simulink model "MyPowerSupply_RTW"  (R2022a)
settings: Solver=ode1  StartTime=0.0  StopTime=inf  FixedStep=0.0002  RelTol=1e-3
PreLoadFcn:
  | vehicle = 'Car'; if ~length(which('cmself')), cmenv; end
  | MyPowerSupply_RTW_bus
InitFcn:
  | vehicle = 'Car'; if ~length(which('cmself')), cmenv; end
  | MyPowerSupply_RTW_bus
libraries: CarMaker4SL x3, simulink x2, simulink_need_slupdate x1
Description:
  | CarMaker Plug-in Model Target
settings Model: ModifiedByFormat=IPG  Creator=IPG  LastModifiedBy=IPG
settings SolverCC: AlgebraicLoopSolver=TrustRegion
settings DebuggingCC: UnconnectedInputMsg=warning  UnconnectedOutputMsg=warning  UnconnectedLineMsg=warning  SFMachineParentedDataDiag=warning
settings RTWCC: Description=CarMaker Plug-in Model Target  SystemTargetFile=CarMaker.tlc  TemplateMakefile=CarMaker_unix-win64.tmf  DLArmComputeVersion=19.05
settings CodeAppCC: MaxIdLength=127
settings STFCustomTargetCC: TargetLangStandard=C99 (ISO)  CombineOutputUpdateFcns=on  CodeInterfacePackaging=Reusable function  GRTInterface=off  GenerateAllocFcn=on  SystemTargetFile=CarMaker.tlc
settings GRTTargetCC: ParMdlRefBuildCompliant=off  CompOptLevelCompliant=off  ConcurrentExecutionCompliant=off  MatFileLogging=off  CodeInterfacePackaging=Reusable function  CPPClassGenCompliant=off  GenerateAllocFcn=on  UseToolchainInfoCompliant=off

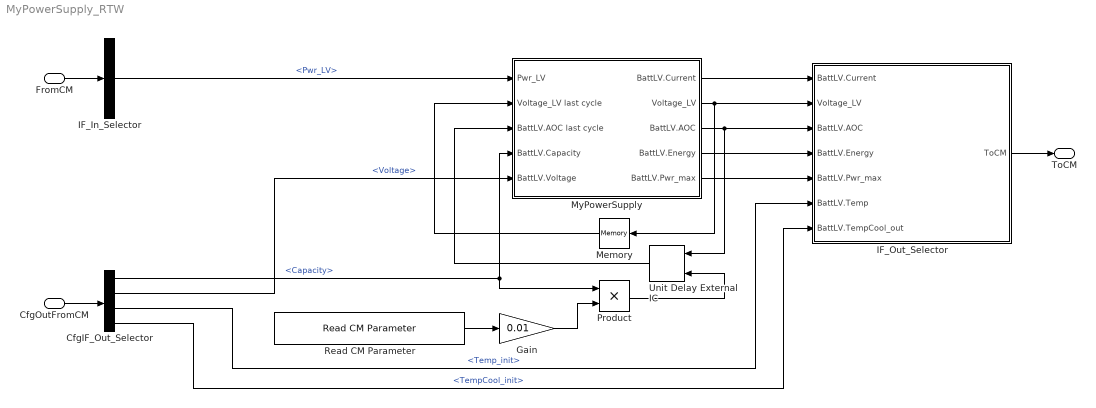
== system MyPowerSupply_RTW ==
  FromCM : Inport  OutDataTypeStr=Bus: cmPTPowerSupplyIn
  CfgOutFromCM : Inport  Port=2  OutDataTypeStr=Bus: cmPTPowerSupplyCfgOut
  CfgIF_Out_Selector : BusSelector  OutputSignals=BattLV.Capacity,BattLV.Voltage,BattLV.Temp_init,BattLV.TempCool_init
  Gain : Gain  Gain=0.01
  IF_In_Selector : BusSelector  OutputSignals=Pwr_LV
  IF_Out_Selector : Subsystem  mask(Signal Selection){}
      mask help: Signal Selection Block
      settings: OpenFcn=cmSignalSelect('SignalSelection_CB',gcb)
  Memory : Memory
  MyPowerSupply : Subsystem
  Product : Product  RndMeth=Zero
  Read CM Parameter : CarMaker4SL/Read CM Parameter  xfile_type=Vehicle  xfile_instance_vehicle=-  xfile_instance_trailer=1  xfile_instance_general=-  xfile_kind_vehicle=Vehicle  xfile_kind_trailer=Trailer  xfile_kind_general=SimParameters  xfile=Vehicle  xkey=PowerTrain.PowerSupply.BattLV.SOC  xnout=1  xdefaults=70.0  xmuxed=on  xstime=Continuous
      settings: SourceProductName=CarMaker4SL
  Unit Delay External IC : simulink_need_slupdate/Unit Delay External IC  tsamp=-1
      settings: SourceProductBaseCode=SL
  ToCM : Outport  OutDataTypeStr=Bus: cmPTPowerSupplyOut
  wires:
  Gain/1 -> Product/2
  CfgIF_Out_Selector/3 -> IF_Out_Selector/6(BattLV.Temp)  "<Temp_init>"
  MyPowerSupply/4(BattLV.Energy) -> IF_Out_Selector/4(BattLV.Energy)
  CfgIF_Out_Selector/1 -> Product/1, MyPowerSupply/4(BattLV.Capacity)  "<Capacity>"
  MyPowerSupply/3(BattLV.AOC) -> Unit Delay External IC/1, IF_Out_Selector/3(BattLV.AOC)
  Read CM Parameter/1 -> Gain/1
  IF_Out_Selector/1(ToCM) -> ToCM/1
  MyPowerSupply/1(BattLV.Current) -> IF_Out_Selector/1(BattLV.Current)
  CfgIF_Out_Selector/2 -> MyPowerSupply/5(BattLV.Voltage)  "<Voltage>"
  IF_In_Selector/1 -> MyPowerSupply/1(Pwr_LV)  "<Pwr_LV>"
  MyPowerSupply/5(BattLV.Pwr_max) -> IF_Out_Selector/5(BattLV.Pwr_max)
  CfgOutFromCM/1 -> CfgIF_Out_Selector/1
  MyPowerSupply/2(Voltage_LV) -> Memory/1, IF_Out_Selector/2(Voltage_LV)
  Memory/1 -> MyPowerSupply/2(Voltage_LV last cycle)
  CfgIF_Out_Selector/4 -> IF_Out_Selector/7(BattLV.TempCool_out)  "<TempCool_init>"
  Unit Delay External IC/1 -> MyPowerSupply/3(BattLV.AOC last cycle)
  FromCM/1 -> IF_In_Selector/1
  Product/1 -> Unit Delay External IC/2

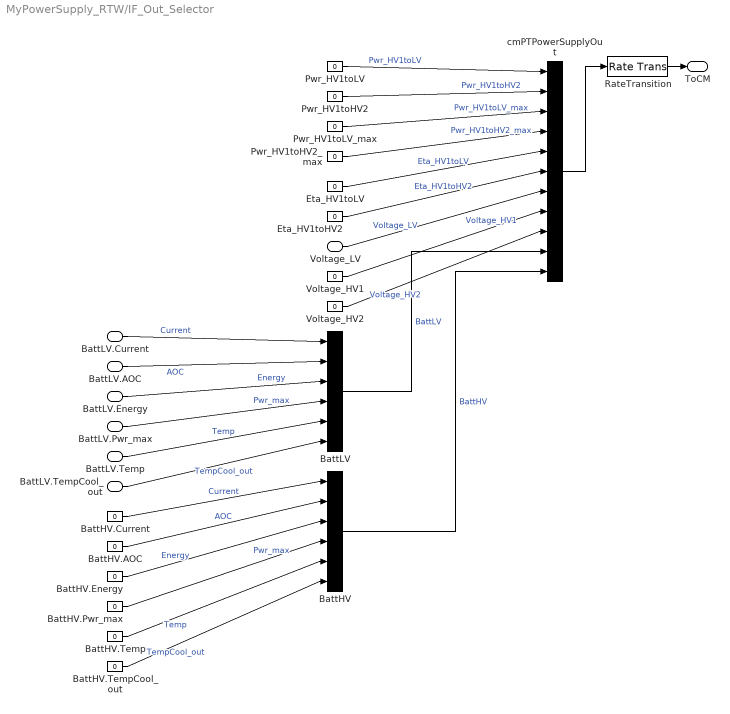
== system MyPowerSupply_RTW/IF_Out_Selector ==
  BattLV.Current : Inport
  Voltage_LV : Inport  Port=2
  BattLV.AOC : Inport  Port=3
  BattLV.Energy : Inport  Port=4
  BattLV.Pwr_max : Inport  Port=5
  BattLV.Temp : Inport  Port=6
  BattLV.TempCool_out : Inport  Port=7
  BattHV : BusCreator  Inputs=6
  BattHV.AOC : Constant  Value=0
  BattHV.Current : Constant  Value=0
  BattHV.Energy : Constant  Value=0
  BattHV.Pwr_max : Constant  Value=0
  BattHV.Temp : Constant  Value=0
  BattHV.TempCool_out : Constant  Value=0
  BattLV : BusCreator  Inputs=6
  Eta_HV1toHV2 : Constant  Value=0
  Eta_HV1toLV : Constant  Value=0
  Pwr_HV1toHV2 : Constant  Value=0
  Pwr_HV1toHV2_max : Constant  Value=0
  Pwr_HV1toLV : Constant  Value=0
  Pwr_HV1toLV_max : Constant  Value=0
  RateTransition : RateTransition  OutPortSampleTime=str2num(get_param(bdroot,'FixedStep'))
  Voltage_HV1 : Constant  Value=0
  Voltage_HV2 : Constant  Value=0
  cmPTPowerSupplyOut : BusCreator  Inputs=11
  ToCM : Outport
  wires:
  RateTransition/1 -> ToCM/1
  cmPTPowerSupplyOut/1 -> RateTransition/1
  Pwr_HV1toLV/1 -> cmPTPowerSupplyOut/1  "Pwr_HV1toLV"
  Pwr_HV1toHV2/1 -> cmPTPowerSupplyOut/2  "Pwr_HV1toHV2"
  Pwr_HV1toLV_max/1 -> cmPTPowerSupplyOut/3  "Pwr_HV1toLV_max"
  Pwr_HV1toHV2_max/1 -> cmPTPowerSupplyOut/4  "Pwr_HV1toHV2_max"
  Eta_HV1toLV/1 -> cmPTPowerSupplyOut/5  "Eta_HV1toLV"
  Eta_HV1toHV2/1 -> cmPTPowerSupplyOut/6  "Eta_HV1toHV2"
  Voltage_HV1/1 -> cmPTPowerSupplyOut/8  "Voltage_HV1"
  Voltage_HV2/1 -> cmPTPowerSupplyOut/9  "Voltage_HV2"
  BattLV/1 -> cmPTPowerSupplyOut/10  "BattLV"
  BattHV/1 -> cmPTPowerSupplyOut/11  "BattHV"
  BattHV.Current/1 -> BattHV/1  "Current"
  BattHV.AOC/1 -> BattHV/2  "AOC"
  BattHV.Energy/1 -> BattHV/3  "Energy"
  BattHV.Pwr_max/1 -> BattHV/4  "Pwr_max"
  BattHV.Temp/1 -> BattHV/5  "Temp"
  BattHV.TempCool_out/1 -> BattHV/6  "TempCool_out"
  BattLV.Current/1 -> BattLV/1  "Current"
  Voltage_LV/1 -> cmPTPowerSupplyOut/7  "Voltage_LV"
  BattLV.AOC/1 -> BattLV/2  "AOC"
  BattLV.Energy/1 -> BattLV/3  "Energy"
  BattLV.Pwr_max/1 -> BattLV/4  "Pwr_max"
  BattLV.Temp/1 -> BattLV/5  "Temp"
  BattLV.TempCool_out/1 -> BattLV/6  "TempCool_out"

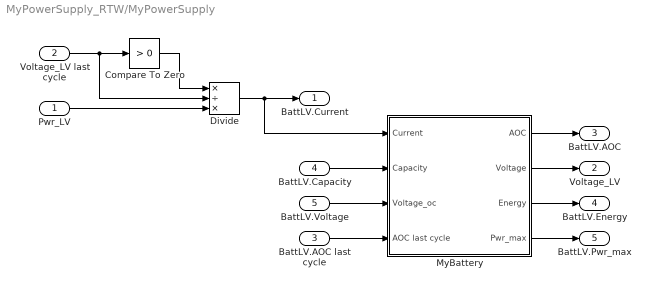
== system MyPowerSupply_RTW/MyPowerSupply ==
  Pwr_LV : Inport
  Voltage_LV last cycle : Inport  Port=2
  BattLV.AOC last cycle : Inport  Port=3
  BattLV.Capacity : Inport  Port=4
  BattLV.Voltage : Inport  Port=5
  Compare To Zero : simulink/Logic and Bit Operations/Compare To Zero  relop=>  OutDataTypeStr=uint8  ZeroCross=off
  Divide : Product  Inputs=*/*
  MyBattery : Subsystem
  BattLV.Current : Outport  VectorParamsAs1DForOutWhenUnconnected=off
  Voltage_LV : Outport  Port=2  VectorParamsAs1DForOutWhenUnconnected=off
  BattLV.AOC : Outport  Port=3  VectorParamsAs1DForOutWhenUnconnected=off
  BattLV.Energy : Outport  Port=4  VectorParamsAs1DForOutWhenUnconnected=off
  BattLV.Pwr_max : Outport  Port=5  VectorParamsAs1DForOutWhenUnconnected=off
  wires:
  Compare To Zero/1 -> Divide/1
  Pwr_LV/1 -> Divide/3
  BattLV.Capacity/1 -> MyBattery/2(Capacity)
  BattLV.Voltage/1 -> MyBattery/3(Voltage_oc)
  BattLV.AOC last cycle/1 -> MyBattery/4(AOC last cycle)
  MyBattery/2(Voltage) -> Voltage_LV/1
  MyBattery/3(Energy) -> BattLV.Energy/1
  MyBattery/4(Pwr_max) -> BattLV.Pwr_max/1
  MyBattery/1(AOC) -> BattLV.AOC/1
  Divide/1 -> BattLV.Current/1, MyBattery/1(Current)
  Voltage_LV last cycle/1 -> Compare To Zero/1, Divide/2

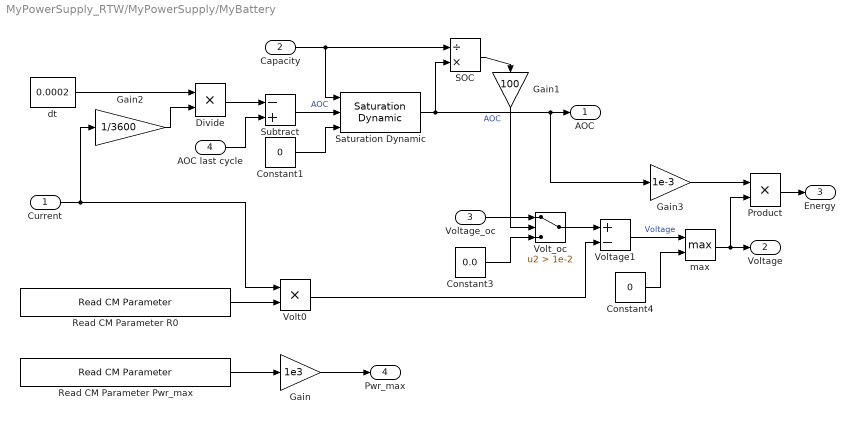
== system MyPowerSupply_RTW/MyPowerSupply/MyBattery ==
  Current : Inport
  Capacity : Inport  Port=2
  Voltage_oc : Inport  Port=3
  AOC last cycle : Inport  Port=4
  Constant1 : Constant  Value=0
  Constant3 : Constant  Value=0.0
  Constant4 : Constant  Value=0
  Divide : Product  Inputs=**
  Gain : Gain  Gain=1e3
  Gain1 : Gain  Gain=100
  Gain2 : Gain  Gain=1/3600
  Gain3 : Gain  Gain=1e-3
  Product : Product  RndMeth=Zero
  Read CM Parameter Pwr_max : CarMaker4SL/Read CM Parameter  xfile=Vehicle  xkey=PowerTrain.PowerSupply.BattLV.Pwr_max  xnout=1  xdefaults=100  xmuxed=on  xstime=Continuous
      settings: SourceProductName=CarMaker4SL
  Read CM Parameter R0 : CarMaker4SL/Read CM Parameter  xfile=Vehicle  xkey=PowerTrain.PowerSupply.BattLV.R0  xnout=1  xdefaults=0.0012  xmuxed=on  xstime=Continuous
      settings: SourceProductName=CarMaker4SL
  SOC : Product  Inputs=/*
  Saturation Dynamic : simulink/Discontinuities/Saturation Dynamic  OutMin=[]  OutMax=[]  OutDataTypeStr=Inherit: Same as second input  OutDataType=sfix(16)  OutScaling=2^-10  DoSatur=off
  Subtract : Sum  Inputs=-+
  Volt0 : Product  RndMeth=Zero
  Volt_oc : Switch  Criteria=u2 > Threshold  Threshold=1e-2  SaturateOnIntegerOverflow=off  InputSameDT=off
  Voltage1 : Sum  Inputs=+-
  dt : Constant  Value=0.0002
  max : MinMax  Function=max  Inputs=2
  AOC : Outport  VectorParamsAs1DForOutWhenUnconnected=off
  Voltage : Outport  Port=2  VectorParamsAs1DForOutWhenUnconnected=off
  Energy : Outport  Port=3  VectorParamsAs1DForOutWhenUnconnected=off
  Pwr_max : Outport  Port=4  VectorParamsAs1DForOutWhenUnconnected=off
  wires:
  Saturation Dynamic/1 -> AOC/1, Gain3/1, SOC/2  "AOC"
  Divide/1 -> Subtract/1
  dt/1 -> Divide/1
  Subtract/1 -> Saturation Dynamic/2  "AOC"
  Constant1/1 -> Saturation Dynamic/3
  Capacity/1 -> Saturation Dynamic/1, SOC/1
  Read CM Parameter Pwr_max/1 -> Gain/1
  SOC/1 -> Gain1/1
  Voltage_oc/1 -> Volt_oc/1
  Constant3/1 -> Volt_oc/3
  Read CM Parameter R0/1 -> Volt0/2
  Volt_oc/1 -> Voltage1/1
  Volt0/1 -> Voltage1/2
  Voltage1/1 -> max/1  "Voltage"
  Constant4/1 -> max/2
  max/1 -> Voltage/1, Product/2
  Product/1 -> Energy/1
  Gain/1 -> Pwr_max/1
  AOC last cycle/1 -> Subtract/2
  Gain2/1 -> Divide/2
  Gain3/1 -> Product/1
  Gain1/1 -> Volt_oc/2
  Current/1 -> Volt0/1, Gain2/1
